simulink model "UFR_Controller_TestSeq_Harness"  (R2023a)
settings: Solver=FixedStepDiscrete  StartTime=0.0  StopTime=5  FixedStep=0.01  RelTol=1e-3
settings Model: Creator=ppatel  LastModifiedBy=ppatel
settings DataIOCC: SaveOutput=off  SaveTime=off
settings OptimizationCC: DefaultParameterBehavior=Inlined  UseDivisionForNetSlopeComputation=on  GainParamInheritBuiltInType=on  UseFloatMulNetSlope=on  InlineInvariantSignals=on  PassReuseOutputArgsAs=Individual arguments  ZeroExternalMemoryAtStartup=off  ZeroInternalMemoryAtStartup=off  NoFixptDivByZeroProtection=on  EfficientFloat2IntCast=on  LifeSpan=1  OptimizeBlockOrder=speed  DifferentSizesBufferReuse=on  EfficientTunableParamExpr=on
settings DebuggingCC: ParameterTunabilityLossMsg=error  SubsystemReferenceDiagnosticForUnitTest=warning
settings HardwareCC: ProdBitPerPointer=32  ProdBitPerSizeT=32  ProdBitPerPtrDiffT=32  ProdLargestAtomicInteger=Long  ProdWordSize=32  ProdLongLongMode=on  ProdHWDeviceType=ARM Compatible->ARM 10
settings SFSimCC: MATLABDynamicMemAlloc=off
settings RTWCC: Description=Embedded Coder  SystemTargetFile=ert.tlc  TemplateMakefile=ert_default_tmf
settings CodeAppCC: ForceParamTrailComments=on  IgnoreCustomStorageClasses=off  OperatorAnnotations=on  SimulinkDataObjDesc=on  SFDataObjDesc=on  CustomSymbolStrGlobalVar=rt$N$M  CustomSymbolStrType=$N$M  CustomSymbolStrFcn=$N$M$F  CustomSymbolStrMacro=$N$M  InsertBlockDesc=on
settings ERTTargetCC: TargetLangStandard=C99 (ISO)  GenerateSampleERTMain=on  IncludeMdlTerminateFcn=off  CombineSignalStateStructs=on  SupportAbsoluteTime=off  SupportComplex=off  SupportContinuousTime=on  SupportNonInlinedSFcns=on  InlinedParameterPlacement=NonHierarchical  ERTCustomFileTemplate=example_file_process.tlc  ERTFilePackagingFormat=CompactWithDataFile

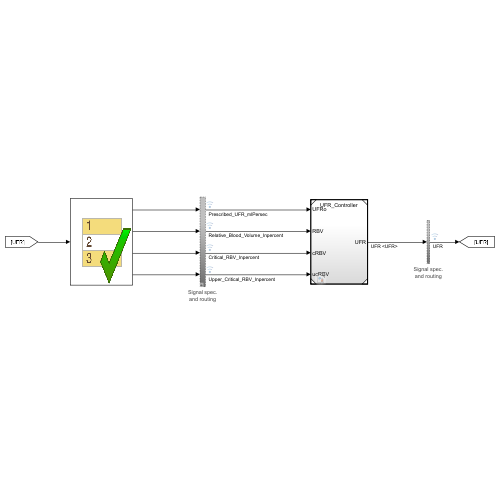
[thumbnail: Simulink's stored preview of the top-level diagram]
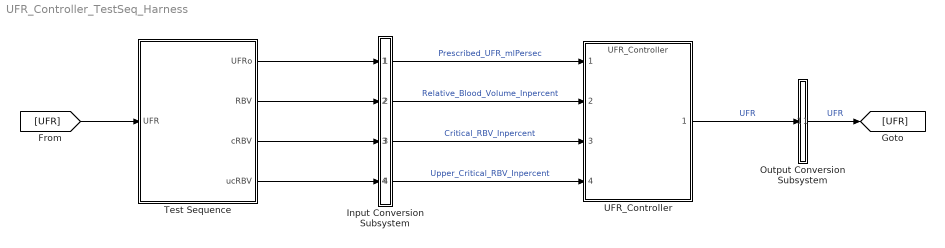
== system UFR_Controller_TestSeq_Harness ==
  Input Conversion Subsystem : Subsystem  Tag=__SLT_ICS__  Description=|
      | Signal spec.
      | and routing
      settings: AttributesFormatString=%<Description>
  Output Conversion Subsystem : Subsystem  Tag=__SLT_OCS__  Description=|
      | Signal spec.
      | and routing
      settings: AttributesFormatString=%<Description>
  Test Sequence : Test Sequence  TreatAsAtomicUnit=on
  UFR_Controller : ModelReference  ModelNameDialog=UFR_Controller  SimulationMode=Normal  ModelReferenceVersion=3.91
  wires:
  Test Sequence/1(UFRo) -> Input Conversion Subsystem/1(Inport_1)
  Test Sequence/2(RBV) -> Input Conversion Subsystem/2(Inport_2)
  Test Sequence/3(cRBV) -> Input Conversion Subsystem/3(Inport_3)
  Test Sequence/4(ucRBV) -> Input Conversion Subsystem/4(Inport_4)
  Output Conversion Subsystem/1(Outport_1) -> [UFR]  "UFR"
  [UFR] -> Test Sequence/1(UFR)
  UFR_Controller/1 -> Output Conversion Subsystem/1(Inport_1)  "UFR"
  Input Conversion Subsystem/1(Outport_1) -> UFR_Controller/1  "Prescribed_UFR_mlPersec"
  Input Conversion Subsystem/2(Outport_2) -> UFR_Controller/2  "Relative_Blood_Volume_Inpercent"
  Input Conversion Subsystem/3(Outport_3) -> UFR_Controller/3  "Critical_RBV_Inpercent"
  Input Conversion Subsystem/4(Outport_4) -> UFR_Controller/4  "Upper_Critical_RBV_Inpercent"

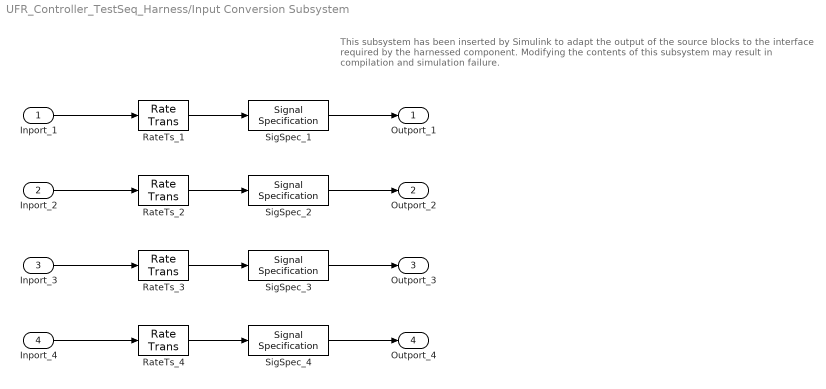
== system UFR_Controller_TestSeq_Harness/Input Conversion Subsystem ==
  note: This subsystem has been inserted by Simulink to adapt the output of the source blocks to the interface required by the harnessed component.
      |  Modifying the contents of this subsystem may result in compilation and simulation failure.
  Inport_1 : Inport
  Inport_2 : Inport  Port=2
  Inport_3 : Inport  Port=3
  Inport_4 : Inport  Port=4
  RateTs_{1..4} (4 alike) : RateTransition  OutPortSampleTime=0.01
  SigSpec_{1..4} (4 alike) : SignalSpecification  OutDataTypeStr=double  Dimensions=[1]  SampleTime=0.01
  Outport_1 : Outport
  Outport_2 : Outport  Port=2
  Outport_3 : Outport  Port=3
  Outport_4 : Outport  Port=4
  wires:
  SigSpec_1/1 -> Outport_1/1
  RateTs_1/1 -> SigSpec_1/1
  Inport_1/1 -> RateTs_1/1
  SigSpec_2/1 -> Outport_2/1
  RateTs_2/1 -> SigSpec_2/1
  Inport_2/1 -> RateTs_2/1
  SigSpec_3/1 -> Outport_3/1
  RateTs_3/1 -> SigSpec_3/1
  Inport_3/1 -> RateTs_3/1
  SigSpec_4/1 -> Outport_4/1
  RateTs_4/1 -> SigSpec_4/1
  Inport_4/1 -> RateTs_4/1

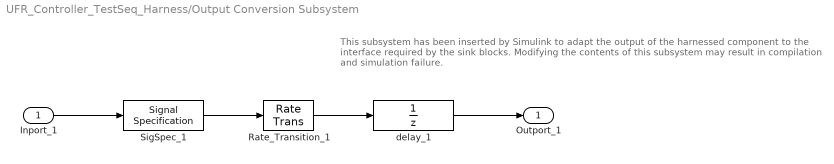
== system UFR_Controller_TestSeq_Harness/Output Conversion Subsystem ==
  note: This subsystem has been inserted by Simulink to adapt the output of the harnessed component to the interface required by the sink blocks.
      |  Modifying the contents of this subsystem may result in compilation and simulation failure.
  Inport_1 : Inport
  Rate_Transition_1 : RateTransition  OutPortSampleTimeOpt=Inherit
  SigSpec_1 : SignalSpecification  OutDataTypeStr=double  Dimensions=[1]  SampleTime=0.01
  delay_1 : UnitDelay  SampleTime=-1
  Outport_1 : Outport
  wires:
  Inport_1/1 -> SigSpec_1/1
  SigSpec_1/1 -> Rate_Transition_1/1
  Rate_Transition_1/1 -> delay_1/1
  delay_1/1 -> Outport_1/1

== stateflow chart UFR_Controller_TestSeq_Harness/Test Sequence ==
  state Constant_UFR
    state Initialize
      %% Initialize data outputs.
      UFRo = 0.18;
      RBV = 100; % Full volume
      cRBV = 94;
      ucRBV = 97;
    state Constant_UFR_Check
      UFRo = 0.18;
      RBV = 100; % Full volume
      state RBV_Reduction
        RBV = 100-ramp(et/0.1);
      (default) -> Constant_UFR.Constant_UFR_Check.RBV_Reduction
    state Verify_NoUFR_Change
      verify(UFR == UFRo);
    state End
    (default) -> Constant_UFR.Initialize
    Constant_UFR.Initialize -> Constant_UFR_Check : [
        | true
        | ]
    Constant_UFR_Check -> Verify_NoUFR_Change : [
        | after(0.2,sec)
        | ]
    Verify_NoUFR_Change -> Constant_UFR.End : [
        | true
        | ]
  state UFR_Adjustment
    state Initialize
      %% Initialize data outputs.
      UFRo = 0.18;
      RBV = 100; % Full volume
      cRBV = 94;
      ucRBV = 97;
    state UFR_Adjustment_Check
      UFRo = 0.18;
      RBV = 100; % Full volume
      state RBV_Reduction
        RBV = 100-ramp(et/0.1);
      (default) -> UFR_Adjustment.UFR_Adjustment_Check.RBV_Reduction
    state Verify_UFR_Reduction
      verify(UFR < UFRo);
    state End
    (default) -> UFR_Adjustment.Initialize
    UFR_Adjustment.Initialize -> UFR_Adjustment_Check : [
        | true
        | ]
    UFR_Adjustment_Check -> Verify_UFR_Reduction : [
        | after(0.4,sec)
        | ]
    Verify_UFR_Reduction -> UFR_Adjustment.End : [
        | true
        | ]
  state UFR_Stop
    state Initialize
      %% Initialize data outputs.
      UFRo = 0.18;
      RBV = 100; % Full volume
      cRBV = 94;
      ucRBV = 97;
    state UFR_Stop_Check
      UFRo = 0.18;
      RBV = 100; % Full volume
      state RBV_Reduction
        RBV = 100-ramp(et/0.1);
      (default) -> UFR_Stop.UFR_Stop_Check.RBV_Reduction
    state Verify_Zero_UFR
      verify(UFR == 0);
    state End
    (default) -> UFR_Stop.Initialize
    UFR_Stop_Check -> Verify_Zero_UFR : [
        | after(0.7,sec)
        | ]
    Verify_Zero_UFR -> UFR_Stop.End : [
        | true
        | ]
    UFR_Stop.Initialize -> UFR_Stop_Check : [
        | true
        | ]
  (default) -> Constant_UFR [order 1] : [Active_Scenario_Index == 1]
  (default) -> UFR_Adjustment [order 2] : [Active_Scenario_Index == 2]
  (default) -> UFR_Stop [order 3] : {assert(Active_Scenario_Index == 3,'The value of Scenario Parameter ''Active_Scenario_Index'' is not valid. Use the index of the scenario to specify it.')}
  data: UFRo output double size=[1]; RBV output double size=[1]; cRBV output double size=[1]; ucRBV output double size=[1]; UFR input; Active_Scenario_Index parameter =1
